simulink model "webserver_demo"  (Simulink 7.3)
settings: Solver=FixedStepDiscrete  SolverMode=SingleTasking  StartTime=0.0  StopTime=10.0  RelTol=1e-3
PreLoadFcn:
  | waijung.modelPreload; % Required for working with Waijung Blockset. Do not remove.
undefined symbols (not defined in the file): A1, A2, A7, B10, B11, B12, Blocking, C1, C2, C3, C4, C5, G14, GPIO_Pin_13, H2, H3, H6, H7, HSEOSC, Link, LQFP176, Non, ST, STM32F417IG
libraries: simulink x14, stm32f4_io_lib x4, waijung_webserver x3, amg_sqlite_dataserver x3, stm32f4_adc_lib x1, stm32f4_device_config_lib x1
(part 1 of 3)
CloseFcn:
  | waijung.modelClose; % Required for working with Waijung Blockset. Do not remove.
settings Model: Creator=Krisada  LastModifiedBy=Krisada
settings OptimizationCC: OptimizeModelRefInitCode=on  LifeSpan=1
settings DebuggingCC: Int32ToFloatConvMsg=none  ParameterPrecisionLossMsg=none
settings HardwareCC: ProdEndianess=LittleEndian  ProdHWDeviceType=ARM Compatible->Cortex - M4  TargetEndianess=LittleEndian  TargetHWDeviceType=ARM Compatible->Cortex - M4
settings RTWCC: SystemTargetFile=stm32f4.tlc  GenerateMakefile=off  TemplateMakefile=ert_default_tmf  Description=STM32F4 Target  ProcessScript=stm32f4_make_rtw_hook
settings CodeAppCC: IgnoreCustomStorageClasses=off
settings STFCustomTargetCC: ModelReferenceCompliant=off  CombineOutputUpdateFcns=on  ERTCustomFileBanners=on  SupportContinuousTime=off  SupportNonInlinedSFcns=off  SystemTargetFile=stm32f4.tlc
settings ERTTargetCC: MultiwordLength=2048  ModelReferenceCompliant=off  ParMdlRefBuildCompliant=off  CompOptLevelCompliant=off  ERTFirstTimeCompliant=off  ModelStepFunctionPrototypeControlCompliant=off  CPPClassGenCompliant=off  ExtModeMexFile=noextcomm  InlinedParameterPlacement=NonHierarchical  ERTSrcFileBannerTemplate=stm32f4_code_template.cgt  ERTHdrFileBannerTemplate=stm32f4_code_template.cgt  ERTDataSrcFileTemplate=stm32f4_code_template.cgt  ERTDataHdrFileTemplate=stm32f4_code_template.cgt  ERTCustomFileTemplate=stm32f4_file_process.tlc

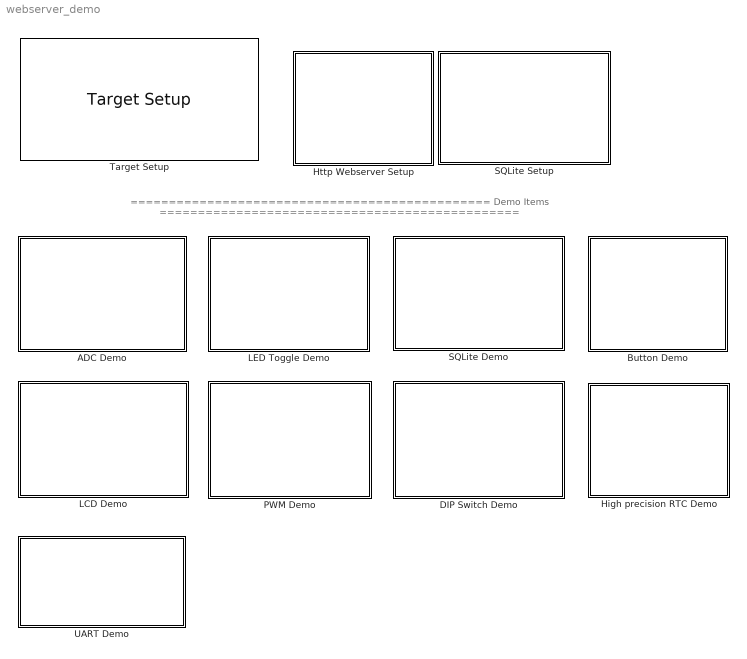
== system webserver_demo ==
  note: =============================================== Demo Items ===============================================
  ADC Demo : Subsystem
  Button Demo : Subsystem
  DIP Switch Demo : Subsystem
  High precision RTC Demo : Subsystem
  Http Webserver Setup : Subsystem
  LCD Demo : Subsystem
  LED Toggle Demo : Subsystem
  PWM Demo : Subsystem
  SQLite Demo : Subsystem
  SQLite Setup : Subsystem
  Target Setup : stm32f4_device_config_lib/Target Setup  Priority=100  compiler=GNU ARM  previous_compiler=GNU ARM  mcu=STM32F417IG (LQFP176)  mcustr=STM32F417IG  clockconfig=HSEOSC-8MHz  system_stm32f4xx_c_path=F:\trunk\targets\stm32f4_target\stm32f4\utils\system_stm32f4xx_default\STM32F40_41xxx\hseosc8mhz  showmemoryconfiguration=on  stacksize=0x2000  heapsize=0x2000  enableautocompiledownload=on  fullchiperase=on  programmerinterface=ST-Link  editctrlstr=on  compilercontrolstr=$(patsubst %, -I%, .) -mcpu=cortex-m4 -mthumb -mthumb-interwork -mfloat-abi=hard -mfpu=fpv4-sp-d16 -ffast-math -Wall -Wextra -Ofast  assemblercontrolstr=$(patsubst %, -I%, .) -mcpu=cortex-m4 -mthumb -mthumb-interwork -mfloat-abi=hard -mfpu=fpv4-sp-d16 -ffast-math -Wall -Wextra -Ofast -Wa,-amhls=$(<:.s=.lst) -D__STACK_SIZE=$(STACK_SIZE) -D__HEAP_SIZE=$(HEAP_SIZE)  linkercontrolstr=-T$(LD_SCRIPT) -g -Wl,-Map=$(MAP),--cref,--no-warn-mismatch -mcpu=cortex-m4 -mthumb -mthumb-interwork -mfloat-abi=hard -mfpu=fpv4-sp-d16 -specs=nosys.specs  runafterdownload=on  execprofile=None  profileruart=1  profilerbaud=115200  profilertxpin=D8  profilerinitstr=0.001,168000000,168000,115200,0  manualsetsampletime=off  sampletime=0.001  blockid=TargetSetup  systickreloadvalue=168000  hseval=8000000  lastprofileruart=1  hclk=168000000  flashorigin=0x8000000  flashlength=1024k  ramorigin=0x20000000  ramlength=128k  useextram=off
  UART Demo : Subsystem

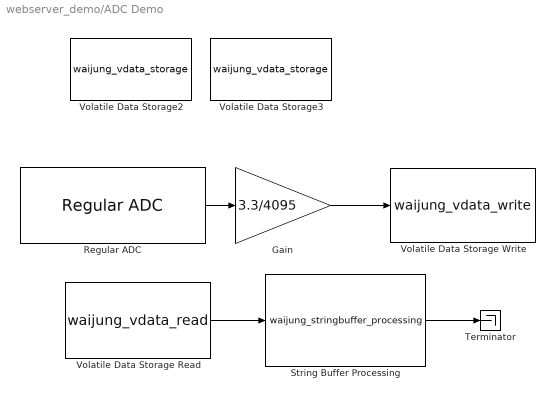
== system webserver_demo/ADC Demo ==
  Gain : Gain  Gain=3.3/4095  ParameterDataTypeMode=single  ParameterDataType=fixdt(1, 16)  ParameterScaling=2^0  ParamDataTypeStr=single  OutDataTypeMode=single  OutDataType=fixdt(1, 16)  OutScaling=2^0  OutDataTypeStr=single
  Regular ADC : stm32f4_adc_lib/Regular ADC  adcmodule=1  outputdatatype=Single  prescaler=2  prescalerstr=ADC_Prescaler_Div2  chsamplingtime=Auto  chsamplingtimestr=ADC_SampleTime_480Cycles  read_an0=off  read_an1=off  read_an2=off  read_an3=off  read_an4=off  read_an5=off  read_an6=off  read_an7=off  read_an8=off  read_an9=off  read_an10=on  read_an11=off  read_an12=off  read_an13=off  read_an14=off  read_an15=off  read_an16=off  read_an17=off  read_an18=off  pinstr=GPIO_Pin_10  usedpinarray="[0  0  0  0  0  0  0  0  0  0  1  0  0  0  0  0  0  0  0]"  usedportidarray=[2]  usedpinidarray=[0]  usedpinidcount=1  sampletime=0.01  blockid=ADCDemoRegularADC  enablecustomportlabel=off  cinputportlabel=0  coutputportlabel=Out1, Out2
  String Buffer Processing : S-Function  FunctionName=waijung_stringbuffer_processing  Parameters=configuration,varname,sformat,porttypes,portcount,inputtypearray,outputtypearray,sampletime,sampletimestr,blockid  EnableBusSupport=off  mask(waijung_stringbuffer_processing){configuration=sprintf, storagename=adc_f, sformat='%1.2f', varname=ADCDemoVolatileDataStorage3_adc_f, inputtypearray=[1 -1], outputtypearray=[1 3], porttypes=["float"], portcount=1, sampletime=-1, sampletimestr=0.001, blockid=ADCDemoStringBufferProcessing}
      mask prompts: configuration "Function"; storagename "String buffer"; sformat "Printf format"; varname "Variable name"; inputtypearray "Input type array"; outputtypearray "Output type array"; porttypes "Port type list"; portcount "Port type count"; sampletime "Sample time (sec)"; sampletimestr "Compiled sample time (sec) in string"
      mask help: This block implements string processing, sprintf/ sscanf command.
      mask init:
      | waijung_stringbuffer_processing_callback('init');
      mask Help: web(fullfile(waijungdocroot,'waijung_stringbuffer_processing.htm'))
      mask StyleString: popup(sprintf|sscanf),popup(adc_f|button_on|button_off|btn2|btn3|btn1|dip|datetime|lcd_line2|lcd_line3|lcd_line4|lcd_line1|<output>),edit,edit,edit,edit,edit,edit,edit,edit,edit
      mask CallbackString: waijung_stringbuffer_processing_callback('configuration');||waijung_stringbuffer_processing_callback('sformat');||||||waijung_stringbuffer_processing_callback('sampletime');|waijung_stringbuffer_processing_callback('sampletimestr');|waijung_stringbuffer_processing_callback('blockid');
      mask Display: text(0.5, 0.5, '[ sprintf ]\nBuffer: adc_f\nTs (sec): 0.001','ver','middle','hor','center');port_label('input', 1,'%f');port_label('output', 1,'Status');
  Terminator : Terminator
  Volatile Data Storage Read : S-Function  FunctionName=waijung_vdata_read  Parameters=storagename,varname,sampletime,sampletimestr,blockid,storagetype,storagetypestr  EnableBusSupport=off  mask(waijung_vdata_read){storagename=adc, varname=ADCDemoVolatileDataStorage2_adc, sampletime=inf, sampletimestr=0.001, blockid=ADCDemoVolatileDataStorageRead, storagetype=single, storagetypestr=float}
      mask prompts: storagename "Storage Name"; varname "Variable name"; sampletime "Sample time (sec)"; sampletimestr "Compiled sample time (sec) in string"; storagetype "Data type"; storagetypestr "Data type string"
      mask help: This block implements read data from a buffer.
      mask init:
      | waijung_vdata_read_callback('init');
      mask Help: web(fullfile(waijungdocroot,'waijung_vdata_read.htm'))
      mask StyleString: popup(adc|adc_f|button_on|button_off|btn2|btn3|btn1|dip|datetime|lcd_line2|lcd_line3|lcd_line4|lcd_line1|led1|pwm),edit,edit,edit,edit,edit,edit
      mask CallbackString: waijung_vdata_read_callback('storagename');|waijung_vdata_read_callback('varname');|waijung_vdata_read_callback('sampletime');|waijung_vdata_read_callback('sampletimestr');|waijung_vdata_read_callback('blockid');|waijung_vdata_read_callback('storagetype');|
      mask Display: text(0.05, 0.5, 'Buffer: adc','ver','middle','hor','left');port_label('output',1,'D1(single)')
  Volatile Data Storage Write : S-Function  FunctionName=waijung_vdata_write  Parameters=storagename,varname,sampletime,sampletimestr,blockid,storagetype,storagetypestr  EnableBusSupport=off  mask(waijung_vdata_write){storagename=adc, varname=ADCDemoVolatileDataStorage2_adc, sampletime=-1, sampletimestr=0.01, blockid=ADCDemoVolatileDataStorageWrite, storagetype=single, storagetypestr=float}
      mask prompts: storagename "Storage Name"; varname "Variable name"; sampletime "Sample time (sec)"; sampletimestr "Compiled sample time (sec) in string"; storagetype "Data type"; storagetypestr "Data type string"
      mask help: This block implements write data to a buffer.
      mask init:
      | waijung_vdata_write_callback('init');
      mask Help: web(fullfile(waijungdocroot,'waijung_vdata_write.htm'))
      mask StyleString: popup(adc|adc_f|button_on|button_off|btn2|btn3|btn1|dip|datetime|lcd_line2|lcd_line3|lcd_line4|lcd_line1|led1|pwm),edit,edit,edit,edit,edit,edit
      mask CallbackString: waijung_vdata_write_callback('storagename');|waijung_vdata_write_callback('varname');|waijung_vdata_write_callback('sampletime');|waijung_vdata_write_callback('sampletimestr');|waijung_vdata_write_callback('blockid');|waijung_vdata_write_callback('storagetype');|
      mask Display: text(0.95, 0.5, 'Buffer: adc','ver','middle','hor','right');port_label('input',1,'D1(single)')
  Volatile Data Storage2 : S-Function  FunctionName=waijung_vdata_storage  Parameters=storagetype,storagename,initval,varname,buffersize,initvalstring,sampletime,sampletimestr,blockid,storagetypestr  EnableBusSupport=off  mask(waijung_vdata_storage){storagetype=single, storagename=adc, initval=0, varname=ADCDemoVolatileDataStorage2_adc, buffersize=64, initvalstring='Initial string', webintegration=ReadOnly, weboutputformat='%1.2f', webcgicallback=(void*)0, sampletime=-1, sampletimestr=0.001, blockid=ADCDemoVolatileDataStorage2, storagetypestr=float}
      mask prompts: storagetype "Storage Type"; storagename "Storage Name (must be a valid variable name)"; initval "Initial value (Apply at Power on Reset only)"; varname "Variable name"; buffersize "Size (bytes)"; initvalstring "Initial value (Apply at Power on Reset only)"; webintegration "Web CGI varget/varset integration"; weboutputformat "Web CGI varget output format"; webcgicallback "Web CGI varset callback"; sampletime "Sample time (sec)"; sampletimestr "Compiled sample time (sec) in string"; storagetypestr "Type string"
      mask help: This block implements a volatile Data Storage.
      mask init:
      | waijung_vdata_storage_callback('init');
      mask Help: web(fullfile(waijungdocroot,'Volatile_Data_Storage.htm'))
      mask StyleString: popup(double|single|uint32|int32|uint16|int16|uint8|int8|string),edit,edit,edit,edit,edit,popup(Disable|ReadOnly|Write/ Read|ReadOnly with KeyValuePair|Write/ Read with KeyValuePair),edit,edit,edit,edit,edit,edit
      mask CallbackString: waijung_vdata_storage_callback('storagetype');|waijung_vdata_storage_callback('storagename');|waijung_vdata_storage_callback('initval');|waijung_vdata_storage_callback('varname');||waijung_vdata_storage_callback('initvalstring');|waijung_vdata_storage_callback('webintegration');|waijung_vdata_storage_callback('weboutputformat');||waijung_vdata_storage_callback('sampletime');|waijung_vdata_storage_callback('sampletimestr');|waijung_vdata_storage_callback('blockid');|
      mask Display: text(0.5, 0.5, 'Name: adc\nType: single','ver','middle','hor','center')
  Volatile Data Storage3 : S-Function  FunctionName=waijung_vdata_storage  Parameters=storagetype,storagename,initval,varname,buffersize,initvalstring,sampletime,sampletimestr,blockid,storagetypestr  EnableBusSupport=off  mask(waijung_vdata_storage){storagetype=string, storagename=adc_f, initval=0, varname=ADCDemoVolatileDataStorage3_adc_f, buffersize=64, initvalstring='', webintegration=ReadOnly, weboutputformat='%s', webcgicallback=(void*)0, sampletime=-1, sampletimestr=0.001, blockid=ADCDemoVolatileDataStorage3, storagetypestr=char}
      mask prompts: storagetype "Storage Type"; storagename "Storage Name (must be a valid variable name)"; initval "Initial value (Apply at Power on Reset only)"; varname "Variable name"; buffersize "Size (bytes)"; initvalstring "Initial value (Apply at Power on Reset only)"; webintegration "Web CGI varget/varset integration"; weboutputformat "Web CGI varget output format"; webcgicallback "Web CGI varset callback"; sampletime "Sample time (sec)"; sampletimestr "Compiled sample time (sec) in string"; storagetypestr "Type string"
      mask help: This block implements a volatile Data Storage.
      mask init:
      | waijung_vdata_storage_callback('init');
      mask Help: web(fullfile(waijungdocroot,'Volatile_Data_Storage.htm'))
      mask StyleString: popup(double|single|uint32|int32|uint16|int16|uint8|int8|string),edit,edit,edit,edit,edit,popup(Disable|ReadOnly|Write/ Read|ReadOnly with KeyValuePair|Write/ Read with KeyValuePair),edit,edit,edit,edit,edit,edit
      mask CallbackString: waijung_vdata_storage_callback('storagetype');|waijung_vdata_storage_callback('storagename');|waijung_vdata_storage_callback('initval');|waijung_vdata_storage_callback('varname');||waijung_vdata_storage_callback('initvalstring');|waijung_vdata_storage_callback('webintegration');|waijung_vdata_storage_callback('weboutputformat');||waijung_vdata_storage_callback('sampletime');|waijung_vdata_storage_callback('sampletimestr');|waijung_vdata_storage_callback('blockid');|
      mask Display: text(0.5, 0.5, 'Name: adc_f\nType: string','ver','middle','hor','center')
  wires:
  Regular ADC/1 -> Gain/1
  String Buffer Processing/1 -> Terminator/1
  Gain/1 -> Volatile Data Storage Write/1
  Volatile Data Storage Read/1 -> String Buffer Processing/1

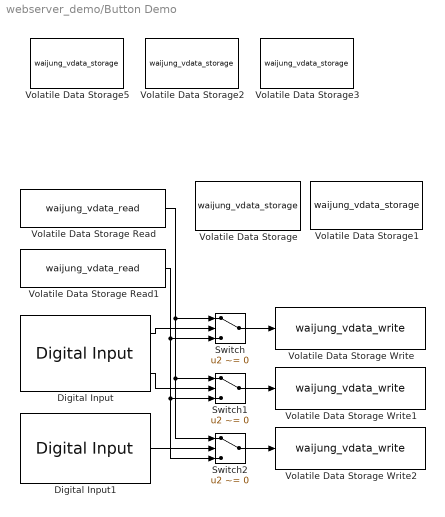
== system webserver_demo/Button Demo ==
  Digital Input : stm32f4_io_lib/Digital Input  port=B  speed=100  porttype=None  porttypestr=NOPULL  use_pin0=off  use_pin1=off  use_pin2=on  use_pin3=off  use_pin4=off  use_pin5=off  use_pin6=off  use_pin7=off  use_pin8=off  use_pin9=off  use_pin10=off  use_pin11=off  use_pin12=off  use_pin13=off  use_pin14=off  use_pin15=on  pinstr=GPIO_Pin_2 | GPIO_Pin_15  usedpinarray="[0  0  1  0  0  0  0  0  0  0  0  0  0  0  0  1]"  bitbandingstr=|  sampletime=0.01  sampletimestr=0.01  blockid=ButtonDemoDigitalInput  enablecustomportlabel=off  glabalinit=off  cinputportlabel=In1, In2  coutputportlabel=Out1, Out2
      | #define ButtonDemoDigitalInput_B2 Peripheral_BB(GPIOB->IDR, 2)  /* Output pin */
      | #define ButtonDemoDigitalInput_B15 Peripheral_BB(GPIOB->IDR, 15)  /* Output pin */
  Digital Input1 : stm32f4_io_lib/Digital Input  port=D  speed=100  porttype=None  porttypestr=NOPULL  use_pin0=off  use_pin1=off  use_pin2=off  use_pin3=off  use_pin4=off  use_pin5=off  use_pin6=off  use_pin7=on  use_pin8=off  use_pin9=off  use_pin10=off  use_pin11=off  use_pin12=off  use_pin13=off  use_pin14=off  use_pin15=off  pinstr=GPIO_Pin_7  usedpinarray="[0  0  0  0  0  0  0  1  0  0  0  0  0  0  0  0]"  bitbandingstr="#define ButtonDemoDigitalInput1_D7 Peripheral_BB(GPIOD->IDR, 7)  /* Output pin */"  sampletime=0.01  sampletimestr=0.01  blockid=ButtonDemoDigitalInput1  enablecustomportlabel=off  glabalinit=off  cinputportlabel=In1, In2  coutputportlabel=Out1, Out2
  Switch : Switch  Criteria=u2 ~= 0  OutDataType=fixdt(1, 16)  OutScaling=2^0
  Switch1 : Switch  Criteria=u2 ~= 0  OutDataType=fixdt(1, 16)  OutScaling=2^0
  Switch2 : Switch  Criteria=u2 ~= 0  OutDataType=fixdt(1, 16)  OutScaling=2^0
  Volatile Data Storage : S-Function  FunctionName=waijung_vdata_storage  Parameters=storagetype,storagename,initval,varname,buffersize,initvalstring,sampletime,sampletimestr,blockid,storagetypestr  EnableBusSupport=off  mask(waijung_vdata_storage){storagetype=string, storagename=button_on, initval=0, varname=ButtonDemoVolatileDataStorage_button_on, buffersize=4, initvalstring='ON', sampletime=-1, sampletimestr=0.001, blockid=ButtonDemoVolatileDataStorage, storagetypestr=char}
      mask prompts: storagetype "Storage Type"; storagename "Storage Name (must be a valid variable name)"; initval "Initial value (Apply at Power on Reset only)"; varname "Variable name"; buffersize "Size (bytes)"; initvalstring "Initial value (Apply at Power on Reset only)"; sampletime "Sample time (sec)"; sampletimestr "Compiled sample time (sec) in string"; storagetypestr "Type string"
      mask help: This block implements a non volatile Data Storage.
      mask init:
      | waijung_vdata_storage_callback('init');
      mask Help: web(fullfile(waijungdocroot,'waijung_vdata_storage.htm'))
      mask StyleString: popup(double|single|uint32|int32|uint16|int16|uint8|int8|string),edit,edit,edit,edit,edit,edit,edit,edit,edit
      mask CallbackString: waijung_vdata_storage_callback('storagetype');|waijung_vdata_storage_callback('storagename');|waijung_vdata_storage_callback('initval');|waijung_vdata_storage_callback('varname');||waijung_vdata_storage_callback('initvalstring');|waijung_vdata_storage_callback('sampletime');|waijung_vdata_storage_callback('sampletimestr');|waijung_vdata_storage_callback('blockid');|
      mask Display: text(0.5, 0.5, '! Out of date','ver','middle','hor','center')
  Volatile Data Storage Read : S-Function  FunctionName=waijung_vdata_read  Parameters=storagename,varname,sampletime,sampletimestr,blockid,storagetype,storagetypestr  EnableBusSupport=off  mask(waijung_vdata_read){storagename=button_on, varname=ButtonDemoVolatileDataStorage_button_on, sampletime=inf, sampletimestr=0.01, blockid=ButtonDemoVolatileDataStorageRead, storagetype=string, storagetypestr=uint32_t}
      mask prompts: storagename "Storage Name"; varname "Variable name"; sampletime "Sample time (sec)"; sampletimestr "Compiled sample time (sec) in string"; storagetype "Data type"; storagetypestr "Data type string"
      mask help: This block implements read data from a buffer.
      mask init:
      | waijung_vdata_read_callback('init');
      mask Help: web(fullfile(waijungdocroot,'waijung_vdata_read.htm'))
      mask StyleString: popup(adc|adc_f|button_on|button_off|btn2|btn3|btn1|dip|datetime|lcd_line2|lcd_line3|lcd_line4|lcd_line1|led1|pwm),edit,edit,edit,edit,edit,edit
      mask CallbackString: waijung_vdata_read_callback('storagename');|waijung_vdata_read_callback('varname');|waijung_vdata_read_callback('sampletime');|waijung_vdata_read_callback('sampletimestr');|waijung_vdata_read_callback('blockid');|waijung_vdata_read_callback('storagetype');|
      mask Display: text(0.05, 0.5, 'Buffer: button_on','ver','middle','hor','left');port_label('output',1,'D1(string)')
  Volatile Data Storage Read1 : S-Function  FunctionName=waijung_vdata_read  Parameters=storagename,varname,sampletime,sampletimestr,blockid,storagetype,storagetypestr  EnableBusSupport=off  mask(waijung_vdata_read){storagename=button_off, varname=ButtonDemoVolatileDataStorage1_button_off, sampletime=inf, sampletimestr=0.01, blockid=ButtonDemoVolatileDataStorageRead1, storagetype=string, storagetypestr=uint32_t}
      mask prompts: storagename "Storage Name"; varname "Variable name"; sampletime "Sample time (sec)"; sampletimestr "Compiled sample time (sec) in string"; storagetype "Data type"; storagetypestr "Data type string"
      mask help: This block implements read data from a buffer.
      mask init:
      | waijung_vdata_read_callback('init');
      mask Help: web(fullfile(waijungdocroot,'waijung_vdata_read.htm'))
      mask StyleString: popup(adc|adc_f|button_on|button_off|btn2|btn3|btn1|dip|datetime|lcd_line2|lcd_line3|lcd_line4|lcd_line1|led1|pwm),edit,edit,edit,edit,edit,edit
      mask CallbackString: waijung_vdata_read_callback('storagename');|waijung_vdata_read_callback('varname');|waijung_vdata_read_callback('sampletime');|waijung_vdata_read_callback('sampletimestr');|waijung_vdata_read_callback('blockid');|waijung_vdata_read_callback('storagetype');|
      mask Display: text(0.05, 0.5, 'Buffer: button_off','ver','middle','hor','left');port_label('output',1,'D1(string)')
  Volatile Data Storage Write : S-Function  FunctionName=waijung_vdata_write  Parameters=storagename,varname,sampletime,sampletimestr,blockid,storagetype,storagetypestr  EnableBusSupport=off  mask(waijung_vdata_write){storagename=btn1, varname=ButtonDemoVolatileDataStorage5_btn1, sampletime=-1, sampletimestr=0.01, blockid=ButtonDemoVolatileDataStorageWrite, storagetype=string, storagetypestr=char*}
      mask prompts: storagename "Storage Name"; varname "Variable name"; sampletime "Sample time (sec)"; sampletimestr "Compiled sample time (sec) in string"; storagetype "Data type"; storagetypestr "Data type string"
      mask help: This block implements write data to a buffer.
      mask init:
      | waijung_vdata_write_callback('init');
      mask Help: web(fullfile(waijungdocroot,'waijung_vdata_write.htm'))
      mask StyleString: popup(adc|adc_f|button_on|button_off|btn2|btn3|btn1|dip|datetime|lcd_line2|lcd_line3|lcd_line4|lcd_line1|led1|pwm),edit,edit,edit,edit,edit,edit
      mask CallbackString: waijung_vdata_write_callback('storagename');|waijung_vdata_write_callback('varname');|waijung_vdata_write_callback('sampletime');|waijung_vdata_write_callback('sampletimestr');|waijung_vdata_write_callback('blockid');|waijung_vdata_write_callback('storagetype');|
      mask Display: text(0.95, 0.5, 'Buffer: btn1','ver','middle','hor','right');port_label('input',1,'D1(string)')
  Volatile Data Storage Write1 : S-Function  FunctionName=waijung_vdata_write  Parameters=storagename,varname,sampletime,sampletimestr,blockid,storagetype,storagetypestr  EnableBusSupport=off  mask(waijung_vdata_write){storagename=btn2, varname=ButtonDemoVolatileDataStorage2_btn2, sampletime=-1, sampletimestr=0.01, blockid=ButtonDemoVolatileDataStorageWrite1, storagetype=string, storagetypestr=char*}
      mask prompts: storagename "Storage Name"; varname "Variable name"; sampletime "Sample time (sec)"; sampletimestr "Compiled sample time (sec) in string"; storagetype "Data type"; storagetypestr "Data type string"
      mask help: This block implements write data to a buffer.
      mask init:
      | waijung_vdata_write_callback('init');
      mask Help: web(fullfile(waijungdocroot,'waijung_vdata_write.htm'))
      mask StyleString: popup(adc|adc_f|button_on|button_off|btn2|btn3|btn1|dip|datetime|lcd_line2|lcd_line3|lcd_line4|lcd_line1|led1|pwm),edit,edit,edit,edit,edit,edit
      mask CallbackString: waijung_vdata_write_callback('storagename');|waijung_vdata_write_callback('varname');|waijung_vdata_write_callback('sampletime');|waijung_vdata_write_callback('sampletimestr');|waijung_vdata_write_callback('blockid');|waijung_vdata_write_callback('storagetype');|
      mask Display: text(0.95, 0.5, 'Buffer: btn2','ver','middle','hor','right');port_label('input',1,'D1(string)')
  Volatile Data Storage Write2 : S-Function  FunctionName=waijung_vdata_write  Parameters=storagename,varname,sampletime,sampletimestr,blockid,storagetype,storagetypestr  EnableBusSupport=off  mask(waijung_vdata_write){storagename=btn3, varname=ButtonDemoVolatileDataStorage3_btn3, sampletime=-1, sampletimestr=0.01, blockid=ButtonDemoVolatileDataStorageWrite2, storagetype=string, storagetypestr=char*}
      mask prompts: storagename "Storage Name"; varname "Variable name"; sampletime "Sample time (sec)"; sampletimestr "Compiled sample time (sec) in string"; storagetype "Data type"; storagetypestr "Data type string"
      mask help: This block implements write data to a buffer.
      mask init:
      | waijung_vdata_write_callback('init');
      mask Help: web(fullfile(waijungdocroot,'waijung_vdata_write.htm'))
      mask StyleString: popup(adc|adc_f|button_on|button_off|btn2|btn3|btn1|dip|datetime|lcd_line2|lcd_line3|lcd_line4|lcd_line1|led1|pwm),edit,edit,edit,edit,edit,edit
      mask CallbackString: waijung_vdata_write_callback('storagename');|waijung_vdata_write_callback('varname');|waijung_vdata_write_callback('sampletime');|waijung_vdata_write_callback('sampletimestr');|waijung_vdata_write_callback('blockid');|waijung_vdata_write_callback('storagetype');|
      mask Display: text(0.95, 0.5, 'Buffer: btn3','ver','middle','hor','right');port_label('input',1,'D1(string)')
  Volatile Data Storage1 : S-Function  FunctionName=waijung_vdata_storage  Parameters=storagetype,storagename,initval,varname,buffersize,initvalstring,sampletime,sampletimestr,blockid,storagetypestr  EnableBusSupport=off  mask(waijung_vdata_storage){storagetype=string, storagename=button_off, initval=0, varname=ButtonDemoVolatileDataStorage1_button_off, buffersize=4, initvalstring='OFF', sampletime=-1, sampletimestr=0.001, blockid=ButtonDemoVolatileDataStorage1, storagetypestr=char}
      mask prompts: storagetype "Storage Type"; storagename "Storage Name (must be a valid variable name)"; initval "Initial value (Apply at Power on Reset only)"; varname "Variable name"; buffersize "Size (bytes)"; initvalstring "Initial value (Apply at Power on Reset only)"; sampletime "Sample time (sec)"; sampletimestr "Compiled sample time (sec) in string"; storagetypestr "Type string"
      mask help: This block implements a non volatile Data Storage.
      mask init:
      | waijung_vdata_storage_callback('init');
      mask Help: web(fullfile(waijungdocroot,'waijung_vdata_storage.htm'))
      mask StyleString: popup(double|single|uint32|int32|uint16|int16|uint8|int8|string),edit,edit,edit,edit,edit,edit,edit,edit,edit
      mask CallbackString: waijung_vdata_storage_callback('storagetype');|waijung_vdata_storage_callback('storagename');|waijung_vdata_storage_callback('initval');|waijung_vdata_storage_callback('varname');||waijung_vdata_storage_callback('initvalstring');|waijung_vdata_storage_callback('sampletime');|waijung_vdata_storage_callback('sampletimestr');|waijung_vdata_storage_callback('blockid');|
      mask Display: text(0.5, 0.5, '! Out of date','ver','middle','hor','center')
  Volatile Data Storage2 : S-Function  FunctionName=waijung_vdata_storage  Parameters=storagetype,storagename,initval,varname,buffersize,initvalstring,sampletime,sampletimestr,blockid,storagetypestr  EnableBusSupport=off  mask(waijung_vdata_storage){storagetype=string, storagename=btn2, initval=0, varname=ButtonDemoVolatileDataStorage2_btn2, buffersize=4, initvalstring='', webintegration=ReadOnly, weboutputformat='%s', webcgicallback=(void*)0, sampletime=-1, sampletimestr=0.001, blockid=ButtonDemoVolatileDataStorage2, storagetypestr=char}
      mask prompts: storagetype "Storage Type"; storagename "Storage Name (must be a valid variable name)"; initval "Initial value (Apply at Power on Reset only)"; varname "Variable name"; buffersize "Size (bytes)"; initvalstring "Initial value (Apply at Power on Reset only)"; webintegration "Web CGI varget/varset integration"; weboutputformat "Web CGI varget output format"; webcgicallback "Web CGI varset callback"; sampletime "Sample time (sec)"; sampletimestr "Compiled sample time (sec) in string"; storagetypestr "Type string"
      mask help: This block implements a volatile Data Storage.
      mask init:
      | waijung_vdata_storage_callback('init');
      mask Help: web(fullfile(waijungdocroot,'Volatile_Data_Storage.htm'))
      mask StyleString: popup(double|single|uint32|int32|uint16|int16|uint8|int8|string),edit,edit,edit,edit,edit,popup(Disable|ReadOnly|Write/ Read|ReadOnly with KeyValuePair|Write/ Read with KeyValuePair),edit,edit,edit,edit,edit,edit
      mask CallbackString: waijung_vdata_storage_callback('storagetype');|waijung_vdata_storage_callback('storagename');|waijung_vdata_storage_callback('initval');|waijung_vdata_storage_callback('varname');||waijung_vdata_storage_callback('initvalstring');|waijung_vdata_storage_callback('webintegration');|waijung_vdata_storage_callback('weboutputformat');||waijung_vdata_storage_callback('sampletime');|waijung_vdata_storage_callback('sampletimestr');|waijung_vdata_storage_callback('blockid');|
      mask Display: text(0.5, 0.5, 'Name: btn2\nType: string','ver','middle','hor','center')
  Volatile Data Storage3 : S-Function  FunctionName=waijung_vdata_storage  Parameters=storagetype,storagename,initval,varname,buffersize,initvalstring,sampletime,sampletimestr,blockid,storagetypestr  EnableBusSupport=off  mask(waijung_vdata_storage){storagetype=string, storagename=btn3, initval=0, varname=ButtonDemoVolatileDataStorage3_btn3, buffersize=4, initvalstring='', webintegration=ReadOnly, weboutputformat='%s', webcgicallback=(void*)0, sampletime=-1, sampletimestr=0.001, blockid=ButtonDemoVolatileDataStorage3, storagetypestr=char}
      mask prompts: storagetype "Storage Type"; storagename "Storage Name (must be a valid variable name)"; initval "Initial value (Apply at Power on Reset only)"; varname "Variable name"; buffersize "Size (bytes)"; initvalstring "Initial value (Apply at Power on Reset only)"; webintegration "Web CGI varget/varset integration"; weboutputformat "Web CGI varget output format"; webcgicallback "Web CGI varset callback"; sampletime "Sample time (sec)"; sampletimestr "Compiled sample time (sec) in string"; storagetypestr "Type string"
      mask help: This block implements a volatile Data Storage.
      mask init:
      | waijung_vdata_storage_callback('init');
      mask Help: web(fullfile(waijungdocroot,'Volatile_Data_Storage.htm'))
      mask StyleString: popup(double|single|uint32|int32|uint16|int16|uint8|int8|string),edit,edit,edit,edit,edit,popup(Disable|ReadOnly|Write/ Read|ReadOnly with KeyValuePair|Write/ Read with KeyValuePair),edit,edit,edit,edit,edit,edit
      mask CallbackString: waijung_vdata_storage_callback('storagetype');|waijung_vdata_storage_callback('storagename');|waijung_vdata_storage_callback('initval');|waijung_vdata_storage_callback('varname');||waijung_vdata_storage_callback('initvalstring');|waijung_vdata_storage_callback('webintegration');|waijung_vdata_storage_callback('weboutputformat');||waijung_vdata_storage_callback('sampletime');|waijung_vdata_storage_callback('sampletimestr');|waijung_vdata_storage_callback('blockid');|
      mask Display: text(0.5, 0.5, 'Name: btn3\nType: string','ver','middle','hor','center')
  Volatile Data Storage5 : S-Function  FunctionName=waijung_vdata_storage  Parameters=storagetype,storagename,initval,varname,buffersize,initvalstring,sampletime,sampletimestr,blockid,storagetypestr  EnableBusSupport=off  mask(waijung_vdata_storage){storagetype=string, storagename=btn1, initval=0, varname=ButtonDemoVolatileDataStorage5_btn1, buffersize=4, initvalstring='', webintegration=ReadOnly, weboutputformat='%s', webcgicallback=(void*)0, sampletime=-1, sampletimestr=0.001, blockid=ButtonDemoVolatileDataStorage5, storagetypestr=char}
      mask prompts: storagetype "Storage Type"; storagename "Storage Name (must be a valid variable name)"; initval "Initial value (Apply at Power on Reset only)"; varname "Variable name"; buffersize "Size (bytes)"; initvalstring "Initial value (Apply at Power on Reset only)"; webintegration "Web CGI varget/varset integration"; weboutputformat "Web CGI varget output format"; webcgicallback "Web CGI varset callback"; sampletime "Sample time (sec)"; sampletimestr "Compiled sample time (sec) in string"; storagetypestr "Type string"
      mask help: This block implements a volatile Data Storage.
      mask init:
      | waijung_vdata_storage_callback('init');
      mask Help: web(fullfile(waijungdocroot,'Volatile_Data_Storage.htm'))
      mask StyleString: popup(double|single|uint32|int32|uint16|int16|uint8|int8|string),edit,edit,edit,edit,edit,popup(Disable|ReadOnly|Write/ Read|ReadOnly with KeyValuePair|Write/ Read with KeyValuePair),edit,edit,edit,edit,edit,edit
      mask CallbackString: waijung_vdata_storage_callback('storagetype');|waijung_vdata_storage_callback('storagename');|waijung_vdata_storage_callback('initval');|waijung_vdata_storage_callback('varname');||waijung_vdata_storage_callback('initvalstring');|waijung_vdata_storage_callback('webintegration');|waijung_vdata_storage_callback('weboutputformat');||waijung_vdata_storage_callback('sampletime');|waijung_vdata_storage_callback('sampletimestr');|waijung_vdata_storage_callback('blockid');|
      mask Display: text(0.5, 0.5, 'Name: btn1\nType: string','ver','middle','hor','center')
  wires:
  Switch/1 -> Volatile Data Storage Write/1
  Volatile Data Storage Read1/1 -> Switch/3, Switch1/3, Switch2/3
  Volatile Data Storage Read/1 -> Switch/1, Switch1/1, Switch2/1
  Digital Input/1 -> Switch/2
  Switch1/1 -> Volatile Data Storage Write1/1
  Digital Input/2 -> Switch1/2
  Switch2/1 -> Volatile Data Storage Write2/1
  Digital Input1/1 -> Switch2/2

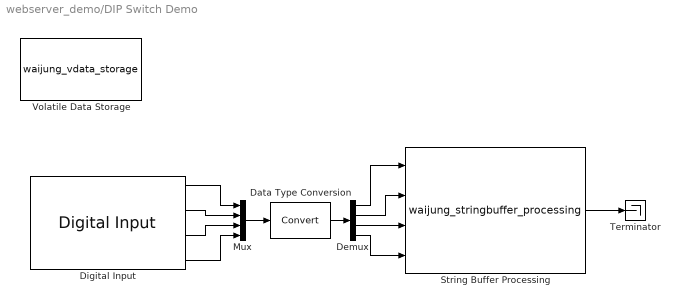
== system webserver_demo/DIP Switch Demo ==
  Data Type Conversion : DataTypeConversion  OutDataType=fixdt(1, 16)  OutScaling=2^0
  Demux : Demux
  Digital Input : stm32f4_io_lib/Digital Input  port=E  speed=100  porttype=None  porttypestr=NOPULL  use_pin0=off  use_pin1=off  use_pin2=off  use_pin3=on  use_pin4=on  use_pin5=on  use_pin6=on  use_pin7=off  use_pin8=off  use_pin9=off  use_pin10=off  use_pin11=off  use_pin12=off  use_pin13=off  use_pin14=off  use_pin15=off  pinstr=GPIO_Pin_3 | GPIO_Pin_4 | GPIO_Pin_5 | GPIO_Pin_6  usedpinarray="[0  0  0  1  1  1  1  0  0  0  0  0  0  0  0  0]"  bitbandingstr=|  sampletime=0.01  sampletimestr=0.01  blockid=DIPSwitchDemoDigitalInput  enablecustomportlabel=off  glabalinit=off  cinputportlabel=In1, In2  coutputportlabel=Out1, Out2
      | #define DIPSwitchDemoDigitalInput_E3 Peripheral_BB(GPIOE->IDR, 3)  /* Output pin */
      | #define DIPSwitchDemoDigitalInput_E4 Peripheral_BB(GPIOE->IDR, 4)  /* Output pin */
      | #define DIPSwitchDemoDigitalInput_E5 Peripheral_BB(GPIOE->IDR, 5)  /* Output pin */
      | #define DIPSwitchDemoDigitalInput_E6 Peripheral_BB(GPIOE->IDR, 6)  /* Output pin */
  Mux : Mux
  String Buffer Processing : S-Function  FunctionName=waijung_stringbuffer_processing  Parameters=configuration,varname,sformat,porttypes,portcount,inputtypearray,outputtypearray,sampletime,sampletimestr,blockid  EnableBusSupport=off  mask(waijung_stringbuffer_processing){configuration=sprintf, storagename=dip, sformat='%u | %u | %u | %u', varname=DIPSwitchDemoVolatileDataStorage_dip, inputtypearray=[4 -1 -1 -1 -1], outputtypearray=[1 3], porttypes=["uint32_t","uint32_t","uint32_t","uint32_t"], portcount=4, sampletime=-1, sampletimestr=0.01, blockid=DIPSwitchDemoStringBufferProcessing}
      mask prompts: configuration "Function"; storagename "String buffer"; sformat "Printf format"; varname "Variable name"; inputtypearray "Input type array"; outputtypearray "Output type array"; porttypes "Port type list"; portcount "Port type count"; sampletime "Sample time (sec)"; sampletimestr "Compiled sample time (sec) in string"
      mask help: This block implements string processing, sprintf/ sscanf command.
      mask init:
      | waijung_stringbuffer_processing_callback('init');
      mask Help: web(fullfile(waijungdocroot,'waijung_stringbuffer_processing.htm'))
      mask StyleString: popup(sprintf|sscanf),popup(adc_f|button_on|button_off|btn2|btn3|btn1|dip|datetime|lcd_line2|lcd_line3|lcd_line4|lcd_line1|<output>),edit,edit,edit,edit,edit,edit,edit,edit,edit
      mask CallbackString: waijung_stringbuffer_processing_callback('configuration');||waijung_stringbuffer_processing_callback('sformat');||||||waijung_stringbuffer_processing_callback('sampletime');|waijung_stringbuffer_processing_callback('sampletimestr');|waijung_stringbuffer_processing_callback('blockid');
      mask Display: text(0.5, 0.5, '[ sprintf ]\nBuffer: dip\nTs (sec): 0.01','ver','middle','hor','center');port_label('input', 1,'%u');port_label('input', 2,'%u');port_label('input', 3,'%u');port_label('input', 4,'%u');port_label('output', 1,'Status');
  Terminator : Terminator
  Volatile Data Storage : S-Function  FunctionName=waijung_vdata_storage  Parameters=storagetype,storagename,initval,varname,buffersize,initvalstring,sampletime,sampletimestr,blockid,storagetypestr  EnableBusSupport=off  mask(waijung_vdata_storage){storagetype=string, storagename=dip, initval=0, varname=DIPSwitchDemoVolatileDataStorage_dip, buffersize=64, initvalstring='', webintegration=Write/ Read, weboutputformat='%s', webcgicallback=(void*)0, sampletime=-1, sampletimestr=0.001, blockid=DIPSwitchDemoVolatileDataStorage, storagetypestr=char}
      mask prompts: storagetype "Storage Type"; storagename "Storage Name (must be a valid variable name)"; initval "Initial value (Apply at Power on Reset only)"; varname "Variable name"; buffersize "Size (bytes)"; initvalstring "Initial value (Apply at Power on Reset only)"; webintegration "Web CGI varget/varset integration"; weboutputformat "Web CGI varget output format"; webcgicallback "Web CGI varset callback"; sampletime "Sample time (sec)"; sampletimestr "Compiled sample time (sec) in string"; storagetypestr "Type string"
      mask help: This block implements a volatile Data Storage.
      mask init:
      | waijung_vdata_storage_callback('init');
      mask Help: web(fullfile(waijungdocroot,'Volatile_Data_Storage.htm'))
      mask StyleString: popup(double|single|uint32|int32|uint16|int16|uint8|int8|string),edit,edit,edit,edit,edit,popup(Disable|ReadOnly|Write/ Read|ReadOnly with KeyValuePair|Write/ Read with KeyValuePair),edit,edit,edit,edit,edit,edit
      mask CallbackString: waijung_vdata_storage_callback('storagetype');|waijung_vdata_storage_callback('storagename');|waijung_vdata_storage_callback('initval');|waijung_vdata_storage_callback('varname');||waijung_vdata_storage_callback('initvalstring');|waijung_vdata_storage_callback('webintegration');|waijung_vdata_storage_callback('weboutputformat');||waijung_vdata_storage_callback('sampletime');|waijung_vdata_storage_callback('sampletimestr');|waijung_vdata_storage_callback('blockid');|
      mask Display: text(0.5, 0.5, 'Name: dip\nType: string','ver','middle','hor','center')
  wires:
  Mux/1 -> Data Type Conversion/1
  Data Type Conversion/1 -> Demux/1
  Digital Input/1 -> Mux/1
  Digital Input/2 -> Mux/2
  Digital Input/3 -> Mux/3
  Digital Input/4 -> Mux/4
  Demux/1 -> String Buffer Processing/1
  Demux/2 -> String Buffer Processing/2
  Demux/3 -> String Buffer Processing/3
  Demux/4 -> String Buffer Processing/4
  String Buffer Processing/1 -> Terminator/1

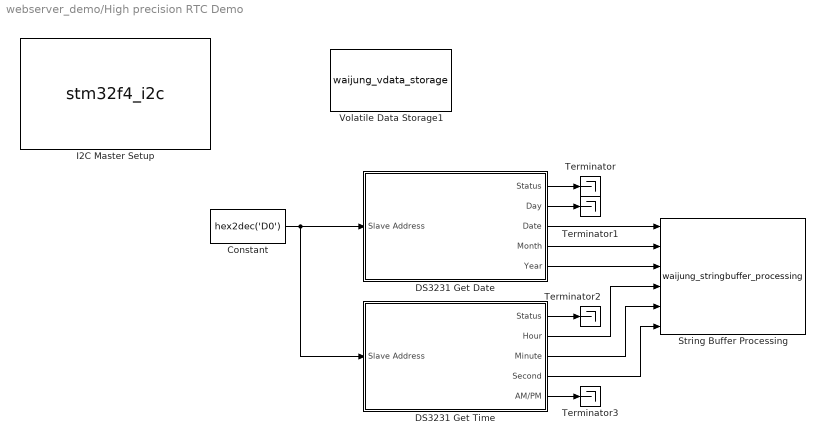
== system webserver_demo/High precision RTC Demo ==
  Constant : Constant  Value=hex2dec('D0')  OutDataTypeMode=uint8  OutDataType=fixdt(1, 16)  OutScaling=2^0  OutDataTypeStr=uint8  SampleTime=1
  DS3231 Get Date : Subsystem  mask{blockfunction=date, module=1}
      mask prompts: blockfunction "Function"; module "I2C module"
      mask init:
      | amg_high_precision_rtc_callback('init');
      mask Help: web(fullfile(waijungdocroot,'DS3231_Get_Date.htm'), '-browser')
      mask StyleString: popup(temp|time|date),popup(1|2|3)
      mask CallbackString: |amg_high_precision_rtc_callback('module');
      mask Display: text(0.5, 0.5, 'Port: I2C1','ver','middle','hor','center');port_label('input', 1,'SlvAddr');port_label('output', 1,'Status');port_label('output', 2,'Day(1-7)');port_label('output', 3,'Date(1-31)');port_label('output', 4,'Month(1-12)');port_label('output', 5,'Year(0-99)');
  DS3231 Get Time : Subsystem  mask{blockfunction=time, module=1}
      mask prompts: blockfunction "Function"; module "I2C module"
      mask init:
      | amg_high_precision_rtc_callback('init');
      mask Help: web(fullfile(waijungdocroot,'DS3231_Get_Time.htm'), '-browser')
      mask StyleString: popup(temp|time|date),popup(1|2|3)
      mask CallbackString: |amg_high_precision_rtc_callback('module');
      mask Display: text(0.5, 0.5, 'Port: I2C1','ver','middle','hor','center');port_label('input', 1,'SlvAddr');port_label('output', 1,'Status');port_label('output', 2,'Hour(0-11/23)');port_label('output', 3,'Minute(0-59)');port_label('output', 4,'Second(0-59)');port_label('output', 5,'AM(0)/PM(1)');
  I2C Master Setup : S-Function  FunctionName=stm32f4_i2c  Parameters=configuration,module,transfer,clkspeed,timeout,sdapin,sclpin,writecount,readcount,inputtypearray,outputtypearray,confstr,sampletime,sampletimestr,blockid  EnableBusSupport=off  mask(stm32f4_i2c){configuration=Setup, module=1, lastmodule=1, transfer=Blocking, dutycycle=TLow/THigh = 2, clkspeed=100, timeout=25, writecount=0, readcount=0, sdapin=B7, sclpin=B6, waitwritetime=0, inputtypearray=[0], outputtypearray=[0], confstr=["B","7","B","6","1","1","6","0","I2C_DutyCycle_2","0","off"], sampletime=-1, sampletimestr=0.001, blockid=HighprecisionRTCDemoI2CMasterSetup}
      mask prompts: module "I2C Module"; lastmodule "Last module"; transfer "Transfer mode"; dutycycle "Duty cycle in fast mode"; clkspeed "Clock speed (kHz)"; timeout "Timeout (ms)"; writecount "Bytes write count"; readcount "Bytes read count"; sdapin "SDA pin"; sclpin "SCL pin"; waitwritetime "Wait write time (ms), default is 0"; inputtypearray "Input type array"; outputtypearray "Output type array"; confstr "Configuration string"; sampletime "Sample time (sec)"; sampletimestr "Compiled sample time (sec) in string"
      mask init:
      | stm32f4_i2c_callback('init');
      mask Help: web(fullfile(waijungdocroot,'stm32f4_i2c_setup.htm'), '-browser')
      mask StyleString: popup(Setup|Transaction),popup(1|2|3),edit,popup(Blocking|Non-blocking),popup(TLow/THigh = 16/9|TLow/THigh = 2),edit,edit,edit,edit,popup(Not used|B7|B9),popup(Not used|B6|B8),edit,edit,edit,edit,edit,edit,edit
      mask CallbackString: stm32f4_i2c_callback('configuration');|stm32f4_i2c_callback('module');|||stm32f4_i2c_callback('dutycycle');|||stm32f4_i2c_callback('writecount');|stm32f4_i2c_callback('readcount');|stm32f4_i2c_callback('sdapin');|stm32f4_i2c_callback('sclpin');||||stm32f4_i2c_callback('confstr');|stm32f4_i2c_callback('sampletime');|stm32f4_i2c_callback('sampletimestr');|stm32f4_i2c_callback('blockid');
      mask Display: text(0.5, 0.5, 'Module: I2C1\nClock: 100kHz\nSDA/SCL Pin: B7/B6','ver','middle','hor','center');
  String Buffer Processing : S-Function  FunctionName=waijung_stringbuffer_processing  Parameters=configuration,varname,sformat,porttypes,portcount,inputtypearray,outputtypearray,sampletime,sampletimestr,blockid  EnableBusSupport=off  mask(waijung_stringbuffer_processing){configuration=sprintf, storagename=datetime, sformat='%u/%u/%u %u:%u:%u', enableoutput=off, varname=HighprecisionRTCDemoVolatileDataStorage1_datetime, inputtypearray=[6 -1 -1 -1 -1 -1 -1], outputtypearray=[0], porttypes=["uint32_t","uint32_t","uint32_t","uint32_t","uint32_t","uint32_t"], portcount=6, sampletime=-1, sampletimestr=1, blockid=HighprecisionRTCDemoStringBufferProcessing}
      mask prompts: configuration "Function"; storagename "String buffer"; sformat "Printf format"; enableoutput "Enable output status"; varname "Variable name"; inputtypearray "Input type array"; outputtypearray "Output type array"; porttypes "Port type list"; portcount "Port type count"; sampletime "Sample time (sec)"; sampletimestr "Compiled sample time (sec) in string"
      mask help:
      | This block implements string processing, sprintf/ sscanf command.
      | Supported format:
      | %u, %i, %o, %x: uint32
      | %d: int32
      | %e, %g, %f: single
      | %c: int8
      |
      | Status:
      |  0: Failed.
      |  Non-zero: Success.
      mask init:
      | waijung_stringbuffer_processing_callback('init');
      mask Help: web(fullfile(waijungdocroot,'String_Buffer_Processing.htm'))
      mask StyleString: popup(sprintf|sscanf),popup(adc_f|button_on|button_off|btn2|btn3|btn1|dip|datetime|lcd_line2|lcd_line3|lcd_line4|lcd_line1|<output>),edit,checkbox,edit,edit,edit,edit,edit,edit,edit,edit
      mask CallbackString: waijung_stringbuffer_processing_callback('configuration');||waijung_stringbuffer_processing_callback('sformat');|waijung_stringbuffer_processing_callback('enableoutput');||||||waijung_stringbuffer_processing_callback('sampletime');|waijung_stringbuffer_processing_callback('sampletimestr');|waijung_stringbuffer_processing_callback('blockid');
      mask Display: text(0.5, 0.5, '[ sprintf ]\nBuffer: datetime\nTs (sec): 1','ver','middle','hor','center');port_label('input', 1,'%u');port_label('input', 2,'%u');port_label('input', 3,'%u');port_label('input', 4,'%u');port_label('input', 5,'%u');port_label('input', 6,'%u');
  Terminator{,1..3} (4 alike) : Terminator
  Volatile Data Storage1 : S-Function  FunctionName=waijung_vdata_storage  Parameters=storagetype,storagename,initval,varname,buffersize,initvalstring,sampletime,sampletimestr,blockid,storagetypestr  EnableBusSupport=off  mask(waijung_vdata_storage){storagetype=string, storagename=datetime, initval=0, varname=HighprecisionRTCDemoVolatileDataStorage1_datetime, buffersize=64, initvalstring='', webintegration=Write/ Read, weboutputformat='%s', webcgicallback=(void*)0, sampletime=-1, sampletimestr=0.001, blockid=HighprecisionRTCDemoVolatileDataStorage1, storagetypestr=char}
      mask prompts: storagetype "Storage Type"; storagename "Storage Name (must be a valid variable name)"; initval "Initial value (Apply at Power on Reset only)"; varname "Variable name"; buffersize "Size (bytes)"; initvalstring "Initial value (Apply at Power on Reset only)"; webintegration "Web CGI varget/varset integration"; weboutputformat "Web CGI varget output format"; webcgicallback "Web CGI varset callback"; sampletime "Sample time (sec)"; sampletimestr "Compiled sample time (sec) in string"; storagetypestr "Type string"
      mask help: This block implements a volatile Data Storage.
      mask init:
      | waijung_vdata_storage_callback('init');
      mask Help: web(fullfile(waijungdocroot,'Volatile_Data_Storage.htm'))
      mask StyleString: popup(double|single|uint32|int32|uint16|int16|uint8|int8|string),edit,edit,edit,edit,edit,popup(Disable|ReadOnly|Write/ Read|ReadOnly with KeyValuePair|Write/ Read with KeyValuePair),edit,edit,edit,edit,edit,edit
      mask CallbackString: waijung_vdata_storage_callback('storagetype');|waijung_vdata_storage_callback('storagename');|waijung_vdata_storage_callback('initval');|waijung_vdata_storage_callback('varname');||waijung_vdata_storage_callback('initvalstring');|waijung_vdata_storage_callback('webintegration');|waijung_vdata_storage_callback('weboutputformat');||waijung_vdata_storage_callback('sampletime');|waijung_vdata_storage_callback('sampletimestr');|waijung_vdata_storage_callback('blockid');|
      mask Display: text(0.5, 0.5, 'Name: datetime\nType: string','ver','middle','hor','center')
  wires:
  Constant/1 -> DS3231 Get Date/1(Slave Address), DS3231 Get Time/1(Slave Address)
  DS3231 Get Date/3(Date) -> String Buffer Processing/1
  DS3231 Get Date/4(Month) -> String Buffer Processing/2
  DS3231 Get Date/5(Year) -> String Buffer Processing/3
  DS3231 Get Time/2(Hour) -> String Buffer Processing/4
  DS3231 Get Time/3(Minute) -> String Buffer Processing/5
  DS3231 Get Time/4(Second) -> String Buffer Processing/6
  DS3231 Get Date/1(Status) -> Terminator/1
  DS3231 Get Date/2(Day) -> Terminator1/1
  DS3231 Get Time/1(Status) -> Terminator2/1
  DS3231 Get Time/5(AM/PM) -> Terminator3/1
